simulink library "posAndVelEstFromLASMeasurements_ul"  (R2020a)
settings: Solver=VariableStepAuto  StartTime=0.0  StopTime=10.0  RelTol=1e-3
settings Model: Creator=jcreed2  LastModifiedBy=andre

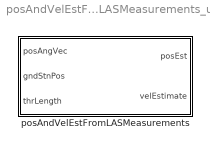
== system posAndVelEstFromLASMeasurements_ul ==
  posAndVelEstFromLASMeasurements : Subsystem

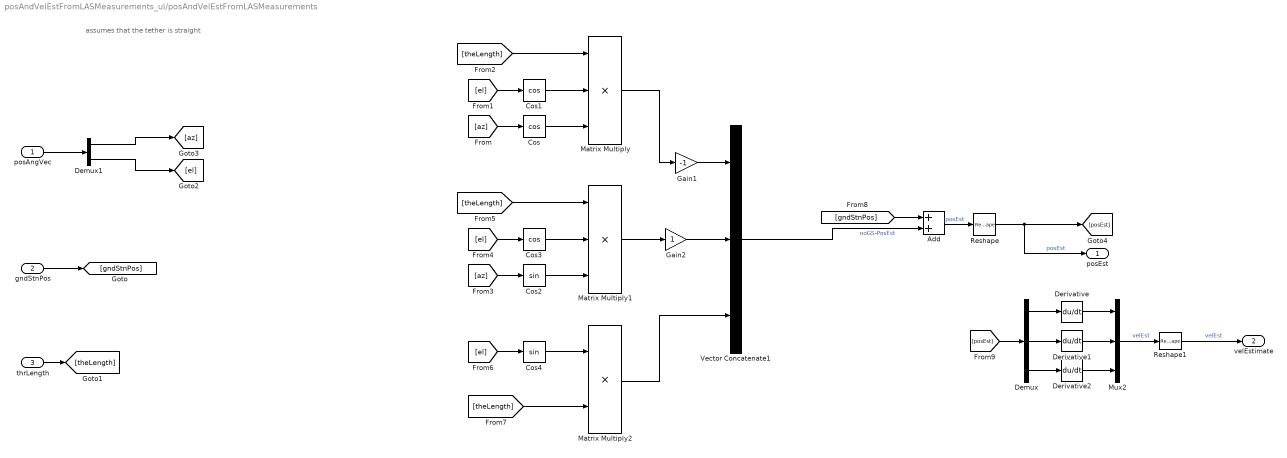
== system posAndVelEstFromLASMeasurements_ul/posAndVelEstFromLASMeasurements ==
  note: assumes that the tether is straight
  posAngVec : Inport
  gndStnPos : Inport  Port=2
  thrLength : Inport  Port=3
  Add : Sum
  Cos : Trigonometry  Operator=cos
  Cos1 : Trigonometry  Operator=cos
  Cos2 : Trigonometry
  Cos3 : Trigonometry  Operator=cos
  Cos4 : Trigonometry
  Demux : Demux  Outputs=3
  Demux1 : Demux  Outputs=2
  Derivative : Derivative
  Derivative1 : Derivative
  Derivative2 : Derivative
  Gain1 : Gain  Gain=-1
  Gain2 : Gain
  Matrix Multiply : Product  Inputs=3
  Matrix Multiply1 : Product  Inputs=3
  Matrix Multiply2 : Product
  Mux2 : Mux  Inputs=3
  Reshape : Reshape  OutputDimensionality=Column vector (2-D)
  Reshape1 : Reshape  OutputDimensionality=Column vector (2-D)
  Vector Concatenate1 : Concatenate  NumInputs=3
  posEst : Outport
  velEstimate : Outport  Port=2
  wires:
  Cos2/1 -> Matrix Multiply1/3
  thrLength/1 -> [theLength]
  [az] -> Cos2/1
  Derivative/1 -> Mux2/1
  Cos/1 -> Matrix Multiply/3
  Demux/3 -> Derivative2/1
  Matrix Multiply/1 -> Gain1/1
  Matrix Multiply1/1 -> Gain2/1
  Reshape/1 -> [posEst], posEst/1  "posEst"
  gndStnPos/1 -> [gndStnPos]
  [theLength] -> Matrix Multiply/1
  Cos1/1 -> Matrix Multiply/2
  [theLength] -> Matrix Multiply2/2
  Demux/2 -> Derivative1/1
  Derivative1/1 -> Mux2/2
  [theLength] -> Matrix Multiply1/1
  [gndStnPos] -> Add/1
  posAngVec/1 -> Demux1/1
  Cos4/1 -> Matrix Multiply2/1
  [el] -> Cos3/1
  [az] -> Cos/1
  Vector Concatenate1/1 -> Add/2  "noGS-PosEst"
  [el] -> Cos4/1
  Cos3/1 -> Matrix Multiply1/2
  Matrix Multiply2/1 -> Vector Concatenate1/3
  [el] -> Cos1/1
  Mux2/1 -> Reshape1/1  "velEst"
  Demux/1 -> Derivative/1
  Derivative2/1 -> Mux2/3
  [posEst] -> Demux/1
  Demux1/2 -> [el]
  Add/1 -> Reshape/1  "posEst"
  Reshape1/1 -> velEstimate/1  "velEst"
  Gain1/1 -> Vector Concatenate1/1
  Gain2/1 -> Vector Concatenate1/2
  Demux1/1 -> [az]
